simulink model "Project9"  (R2025b)
settings: Solver=ode23t  StartTime=0.0  StopTime=0.1  RelTol=1e-3
libraries: ee_lib x5, nesl_utility x5, fl_lib x4, eePwmGenerator x1
settings Model: Creator=mertc  LastModifiedBy=mertc

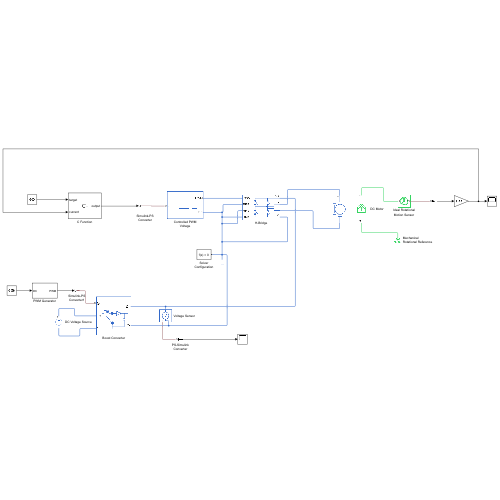
[thumbnail: Simulink's stored preview of the top-level diagram]
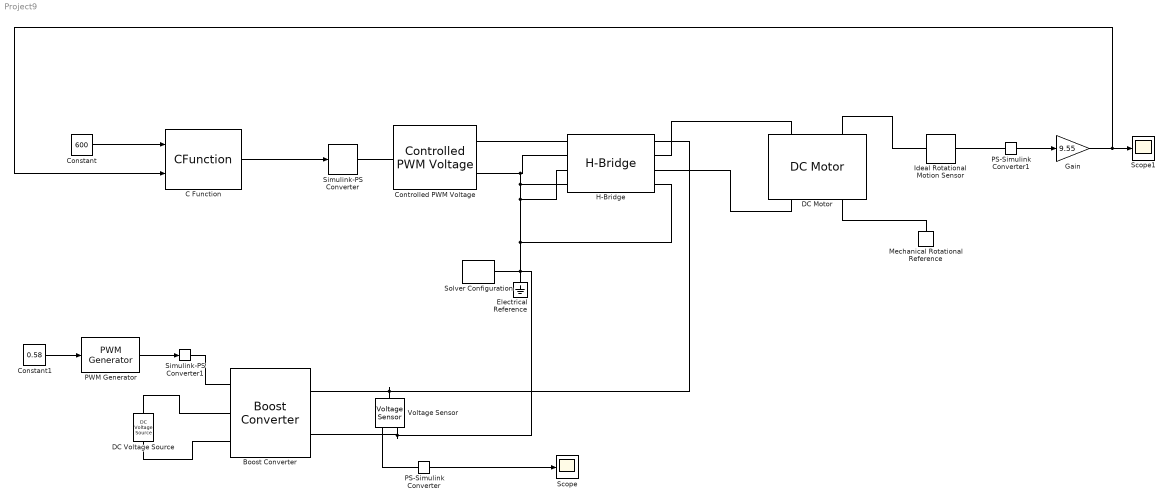
== system Project9 ==
  Boost Converter : ee_lib/Semiconductors & Converters/Converters/Boost Converter  port_option=ee.enum.controlport.ps  device_type=ee.enum.converters.switchingdevice.ideal  Vf=0.8 V  Ron=0.001 Ohm  Rds=0.001 Ohm  Goff=1e-5 1/Ohm  Vgt=1 V  Vgt_off=-1 V  Ih=1 A  Vth=0.5 V  K=0  diode_param=ee.enum.converters.diode.nodynamics  diode_Vf=0.4 V  diode_Ron=0.05 Ohm  diode_Goff=1e-6 1/Ohm  diode_C=50 nF  diode_iRM=-235 A  diode_iF=300 A  diode_idot=-50 A/us  diode_trr_param=ee.enum.converters.diodetrr.trr_factor  diode_trr_factor=3  diode_trr=15 us  diode_Qrr=1500 s*uA  Lf=47e-6 H  Rl=0.1 Ohm  Cf=470e-6 F  Rf=0.01 Ohm  snubber_type=ee.enum.converters.snubber.exclude  Cs=1e-7 F  Rs=0.1 Ohm  iL_specify=off  iL_priority=High  iL=0 A  iL_nominal_specify=off  iL_nominal_value=1  iL_nominal_unit=A  vc_specify=off  vc_priority=High  vc=0 V  vc_nominal_specify=off  vc_nominal_value=1  vc_nominal_unit=V
      settings: InternalSimscapePortConfiguration="{\"Bottom\":[],\"Left\":[{\"id\":\"G\",\"label\":\"G\",\"type\":\"input\"},{\"id\":\"p1\",\"label\":\"1+\",\"type\":\"foundation.electrical.electrical\"},{\"id\":\"n1\",\"label\":\"1-\",\"type\":\"foundation.electrical.electrical\"}],\"Right\":[{\"id\":\"p2\",\"label\":\"2+\",\"type\":\"foundation.electrical.electrical\"},{\"id\":\"n2\",\"label\":\"2-\",\"type\":\"foundation.electrical.electrical\"}],\"Top\":[]}"
  C Function : CFunction  OutputCode=|  CodegenOutputCode=|  SampleTime=0.001  CustomCodeSettingLocation=ModelConfigurationParameters
      OutputCode=|
      | /* Gerçek PI Kontrol Mantığı */
      | float error = u1 - u2;              // u1: Hedef (600), u2: Mevcut RPM
      | float Kp = 0.05f;                   
      | float Ki = 0.2f;                    
      | 
      | // Hataları topla (Simulink hafızasında duran integral_error'ı kullanıyoruz)
      | integral_error += error * 0.001f;   
      | 
      | // Çıkış Gücü
      | y1 = 15.0f + (Kp * error) + (Ki * integral_error);
      | 
      | // Anti-Windup ve Sınırlandırma
      | if (y1 > 100.0f) {
      |     y1 = 100.0f;
      |     integral_error -= error * 0.001f; // Doyumda biriktirmeyi kes
      | }
      | if (y1 < 0.0f) {
      |     y1 = 0.0f;
      |     integral_error -= error * 0.001f;
      | }
      CodegenOutputCode=|
      | /* Gerçek PI Kontrol Mantığı */
      | float error = u1 - u2;              // u1: Hedef (600), u2: Mevcut RPM
      | float Kp = 0.05f;                   
      | float Ki = 0.2f;                    
      | 
      | // Hataları topla (Simulink hafızasında duran integral_error'ı kullanıyoruz)
      | integral_error += error * 0.001f;   
      | 
      | // Çıkış Gücü
      | y1 = 15.0f + (Kp * error) + (Ki * integral_error);
      | 
      | // Anti-Windup ve Sınırlandırma
      | if (y1 > 100.0f) {
      |     y1 = 100.0f;
      |     integral_error -= error * 0.001f; // Doyumda biriktirmeyi kes
      | }
      | if (y1 < 0.0f) {
      |     y1 = 0.0f;
      |     integral_error -= error * 0.001f;
      | }
  Constant : Constant  Value=600
  Constant1 : Constant  Value=0.58
  Controlled PWM Voltage : ee_lib/Integrated Circuits/Controlled PWM Voltage  F=20000 Hz  TD=0 s  pulse_width_offset=0 s  pulse_min=0 s  pwm_or_av=ee.enum.pwm_or_av.pwm  event_type=ee.enum.ic.event.asynchronous  sample_time=1e-6 s  Vmin=0 V  Vmax=5 V  Vm=5 V  u_min=0  u_max=100
      settings: InternalSimscapePortConfiguration="{\"Bottom\":[],\"Left\":[{\"id\":\"u\",\"label\":\"u\",\"type\":\"input\"}],\"Right\":[{\"id\":\"p2\",\"label\":\"PWM\",\"type\":\"foundation.electrical.electrical\"},{\"id\":\"n2\",\"label\":\"REF\",\"type\":\"foundation.electrical.electrical\"}],\"Top\":[]}"
  DC Motor : ee_lib/Electromechanical/Brushed Motors/DC Motor  field_option=ee.enum.field_option.pm  Rf=100 Ohm  Lf=1 H  Laf=0.15 H  If0=0 A  parameterization=ee.enum.dcparam_option.circuit_param  Ra=20 Ohm  La=0.0015 H  emf_or_torque=ee.enum.emf_or_torque.kv  Kv=0.172 V*s/rad  Ki=6.876e-4 N*m/A  T_stall=0.24e-3 N*m  w_max=19100 rpm  w_rated=15000 rpm  P_rated=0.08 W  V_rated=1.5 V  lam_param=ee.enum.lam_param.damping  i_noload=0 A  V_i_noload=1.5 V  J=1e-6 kg*m^2  lam=1e-5 N*m*s/rad  speed0=0 rpm  alpha=3.93e-3 1/K  Tmeas=25 degC  thermal_mass=100 J/K  initial_temperature=25 degC
  DC Voltage Source : ee_lib/Additional Components/SPICE Sources/DC Voltage Source  DC=5 V
  Electrical Reference : fl_lib/Electrical/Electrical Elements/Electrical Reference
  Gain : Gain  Gain=9.55
  H-Bridge : ee_lib/Semiconductors & Converters/Converters/H-Bridge  supply_ports=ee.enum.supply_ports.showsupply  pwm_or_av=ee.enum.pwm_or_av.pwm  regenerative_braking_mode=ee.enum.converters.regenerative_braking_mode.depends_on_rev  discontinuous=ee.enum.current_profile.continuous  freewheeling_mode=ee.enum.converters.freewheeling_mode.one_switch_one_diode  Rload=10 Ohm  Lload=1e-5 H  F=10 kHz  Venable=0.5 V  Vmax=5.0 V  Vreverse=0.5 V  Vbrake=0.5 V  Vm=12 V  Ron=2 Ohm  Don=0.05 Ohm  Goff=1e-6 S  Tmeas=298.15 K  Ron2=0.1 Ohm  Don2=0.05 Ohm  Tmeas2=398.15 K  thermal_mass=100 J/K  initial_temperature=298.15 K
      settings: InternalSimscapePortConfiguration="{\"Bottom\":[],\"Left\":[{\"id\":\"ENA\",\"label\":\"PWM\",\"type\":\"foundation.electrical.electrical\"},{\"id\":\"REF\",\"label\":\"REF\",\"type\":\"foundation.electrical.electrical\"},{\"id\":\"REV\",\"label\":\"REV\",\"type\":\"foundation.electrical.electrical\"},{\"id\":\"BRK\",\"label\":\"BRK\",\"type\":\"foundation.electrical.electrical\"}],\"Right\":[{\"id\":\"p1\",\"label\":\"V+\",\"type\":\"foundation.electrical.electrical\"},{\"id\":\"p2\",\"label\":\"+\",\"type\":\"foundation.electrical.electrical\"},{\"id\":\"n2\",\"label\":\"-\",\"type\":\"foundation.electrical.electrical\"},{\"id\":\"n1\",\"label\":\"V-\",\"type\":\"foundation.electrical.electrical\"}],\"Top\":[]}"
  Ideal Rotational Motion Sensor : fl_lib/Mechanical/Mechanical Sensors/Ideal Rotational Motion Sensor  reference=foundation.enum.MeasurementReference.absolute  acceleration_port=false  velocity_port=true  position_port=false  wrap_angle=false  offset=0 rad
      settings: InternalSimscapePortConfiguration="{\"Bottom\":[],\"Left\":[{\"id\":\"R\",\"label\":\"R\",\"type\":\"foundation.mechanical.rotational.rotational\"}],\"Right\":[{\"id\":\"W\",\"label\":\"W\",\"type\":\"output\"}],\"Top\":[]}"
  Mechanical Rotational Reference : fl_lib/Mechanical/Rotational Elements/Mechanical Rotational Reference
  PS-Simulink Converter : nesl_utility/PS-Simulink Converter  PhysicalDomain=network_engine_domain  SubClassName=ps_output  LeftPortType=input  RightPortType=output  PseudoPeriodic=off  Frequencies=[]  VectorFormat=inherit  Unit=inherit  AffineConversion=off
  PS-Simulink Converter1 : nesl_utility/PS-Simulink Converter  PhysicalDomain=network_engine_domain  SubClassName=ps_output  LeftPortType=input  RightPortType=output  PseudoPeriodic=off  Frequencies=[]  VectorFormat=inherit  Unit=inherit  AffineConversion=off
  PWM Generator : eePwmGenerator/PWM Generator  CarrCount=Up  Tper=0.0000025  Tdelay=0  Ts=0
  Scope : Scope
      settings: ActiveDisplayYMinimum=-1.6866232118058946  ActiveDisplayYMaximum=15.179608906253055
  Scope1 : Scope
      settings: ActiveDisplayYMinimum=-73.2244508662389  ActiveDisplayYMaximum=659.02005779615024
  Simulink-PS Converter : nesl_utility/Simulink-PS Converter  PhysicalDomain=network_engine_domain  SubClassName=ps_input  LeftPortType=input  RightPortType=output  PseudoPeriodic=off  Frequencies=[]  NoiseDistribution=none  NoiseParameters=[]  Unit=1  AffineConversion=off  FilteringAndDerivatives=provide  SimscapeFilterOrder=1  InputFilterTimeConstant=0.001  UdotUserProvided=0
  Simulink-PS Converter1 : nesl_utility/Simulink-PS Converter  PhysicalDomain=network_engine_domain  SubClassName=ps_input  LeftPortType=input  RightPortType=output  PseudoPeriodic=off  Frequencies=[]  NoiseDistribution=none  NoiseParameters=[]  Unit=1  AffineConversion=off  FilteringAndDerivatives=provide  SimscapeFilterOrder=1  InputFilterTimeConstant=0.001  UdotUserProvided=0
  Solver Configuration : nesl_utility/Solver Configuration  PhysicalDomain=network_engine_domain  SubClassName=solver  LeftPortType=input  RightPortType=generic  Tones=[]  Harmonics=[]  SimulateNoise=off  Profile=off  UseLocalSampling=off  EnableSwitchedLinearOptims=on  FrequencyDomain=off  UseCCode=off  RelTol=0.001  AbsTol=0.001  MinStep=1e-09  ToWorkspace=off  RevertToSquareIcSolve=off  NumHomotopyIterations=100  PhasorMode=off  PhasorModeNumHarmonics=1  ConsistencySolver=NEWTON_XTOL_AFTER_FTOL  IndexReductionMethod=DerivativeReplacement  DoDC=off  ResidualTolerance=1e-09  ConsistencyTolSource=GLOBAL  ConsistencyAbsTol=0.001  ConsistencyRelTol=0.001  ConsistencyTolFactor=0.001  UseLocalSolver=off  LocalSolverChoice=NE_BACKWARD_EULER_ADVANCER  ResolveIndetEquations=on  FunctionEvalNumThread=1  LocalSolverSampleTime=0.001  DoFixedCost=off  MaxNonlinIter=3  MaxModeIter=2  ComputeImpulses=off  ImpulseIterations=2  LinearAlgebra=auto  LinearAlgebraNumThread=0  EquationFormulation=NE_TIME_EF  DelaysMemoryBudget=1024  AutomaticFiltering=on  FilteringTimeConstant=0.001  PartitionStorageMethod=AS_NEEDED  PartitionMemoryBudget=1024  PartitionMethod=ROBUST  MultibodyUseLocalSolver=off  MultibodyLocalSolverChoice=ODE1  MultibodyLocalSolverSampleTime=0.001
  Voltage Sensor : fl_lib/Electrical/Electrical Sensors/Voltage Sensor
  wires:
  PWM Generator/1 -> Simulink-PS Converter1/1
  Constant1/1 -> PWM Generator/1
  Gain/1 -> C Function/2, Scope1/1
  PS-Simulink Converter1/1 -> Gain/1
  C Function/1 -> Simulink-PS Converter/1
  PS-Simulink Converter/1 -> Scope/1
  Constant/1 -> C Function/1
  connections:
  H-Bridge/LConn2 -- Controlled PWM Voltage/RConn2 -- Voltage Sensor/RConn2 -- Boost Converter/RConn2 -- Solver Configuration/RConn1 -- Electrical Reference/LConn1 -- H-Bridge/RConn4 -- H-Bridge/LConn3 -- H-Bridge/LConn4
  Boost Converter/RConn1 -- Voltage Sensor/LConn1 -- H-Bridge/RConn1
  DC Voltage Source/RConn1 -- Boost Converter/LConn3
  DC Voltage Source/LConn1 -- Boost Converter/LConn2
  DC Motor/RConn2 -- Mechanical Rotational Reference/LConn1
  DC Motor/LConn2 -- Ideal Rotational Motion Sensor/LConn1
  PS-Simulink Converter/LConn1 -- Voltage Sensor/RConn1
  PS-Simulink Converter1/LConn1 -- Ideal Rotational Motion Sensor/RConn1
  Simulink-PS Converter1/RConn1 -- Boost Converter/LConn1
  H-Bridge/RConn2 -- DC Motor/LConn1
  Controlled PWM Voltage/RConn1 -- H-Bridge/LConn1
  Simulink-PS Converter/RConn1 -- Controlled PWM Voltage/LConn1
  H-Bridge/RConn3 -- DC Motor/RConn1
